simulink subsystem "Actuator_Dynamics"  (R2025b)
settings: Solver=VariableStepAuto  StartTime=0.0  StopTime=10.0  RelTol=1e-3
values from neighbouring files (symbols this model uses):
  Actuator_Delay = 0.01    [data.m]
  Actuator_ServoMaxRate = 270    [data.m]
  Actuator_Tau = 0.05    [data.m]
settings Model: Creator=Filip  LastModifiedBy=Filip

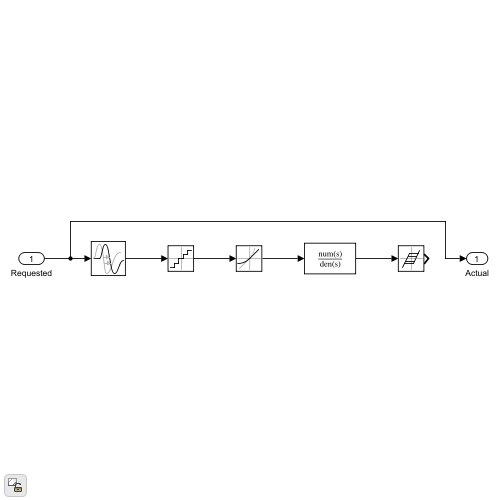
[thumbnail: Simulink's stored preview of the top-level diagram]
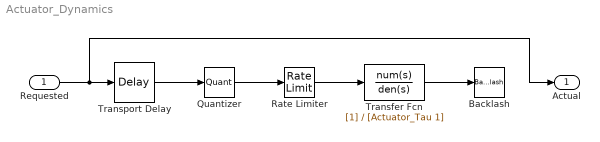
== system Actuator_Dynamics ==
  Requested : Inport
  Backlash : Backlash  BacklashWidth=Actuator_DeadZone  ZeroCross=off
  Quantizer : Quantizer  QuantizationInterval=Actuator_ServoStep
  Rate Limiter : RateLimiter  RisingSlewLimit=+Actuator_ServoMaxRate  FallingSlewLimit=-Actuator_ServoMaxRate  SampleTimeMode=inherited
  Transfer Fcn : TransferFcn  Denominator=[Actuator_Tau 1]
  Transport Delay : TransportDelay  DelayTime=Actuator_Delay
  Actual : Outport
  wires:
  Transport Delay/1 -> Quantizer/1
  Quantizer/1 -> Rate Limiter/1
  Rate Limiter/1 -> Transfer Fcn/1
  Transfer Fcn/1 -> Backlash/1
  Requested/1 -> Transport Delay/1, Actual/1
